simulink model "SimulacionTanque2"  (R2020a)
settings: Solver=VariableStepAuto  StartTime=0.0  StopTime=tsim  RelTol=1e-3
values from neighbouring files (symbols this model uses):
  tmuestra = 0.5    [GeneracionDatosTanque.m]    (also in LQRTanque.m; SimulacionTanque.m)
  tvar1 = 23    [GeneracionDatosTanque.m]    (also in SimulacionTanque.m)
  tvar2 = 24    [GeneracionDatosTanque.m]    (also in SimulacionTanque.m)
undefined symbols (not defined in the file or in its folder): alpha, Area, K1, K2, Kp, T1, T2, tau1, tau2, tdelay1, tdelay2, tdelayQ, Te
settings Model: Creator=pablo  LastModifiedBy=pablo
settings DataIOCC: SaveOutput=off  SignalLogging=off  DSMLogging=off  SaveTime=off  ReturnWorkspaceOutputs=off
settings DebuggingCC: ArithmeticOperatorsInVariantConditions=warning
settings SFSimCC: CustomCodeUndefinedFunction=UseInterfaceOnly

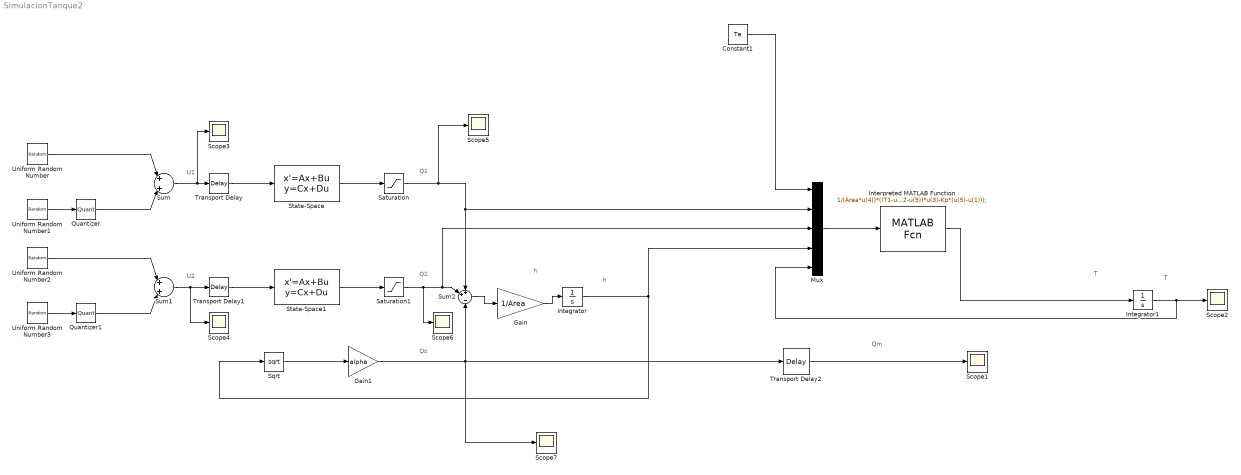
== system SimulacionTanque2 ==
  note: Qm
  note: .
      | T
  note: T
  note: h
  note: .
      |  h
  note: Qs
  note: Q1
  note: U1
  note: Q2
  note: U2
  Constant1 : Constant  Value=Te
  Gain : Gain  Gain=1/Area
  Gain1 : Gain  Gain=alpha
  Integrator : Integrator  InitialCondition=(4/alpha^2)  LimitOutput=on  LowerSaturationLimit=0
  Integrator1 : Integrator  InitialCondition=49.9  LowerSaturationLimit=0
  Interpreted MATLAB Function : MATLABFcn  MATLABFcn=1/(Area*u(4))*((T1-u(5))*u(2)+(T2-u(5))*u(3)-Kp*(u(5)-u(1)));  OutputDimensions=1
  Mux : Mux  Inputs=5
  Quantizer : Quantizer  QuantizationInterval=.25
  Quantizer1 : Quantizer  QuantizationInterval=.25
  Saturation : Saturate  UpperLimit=inf  LowerLimit=0
  Saturation1 : Saturate  UpperLimit=inf  LowerLimit=0
  Scope{1..7} (7 alike) : Scope
  Sqrt : Sqrt  SaturateOnIntegerOverflow=on
  State-Space : StateSpace  A=-1/tau1  B=K1/tau1  D=0  InitialCondition=2
  State-Space1 : StateSpace  A=-1/tau2  B=K2/tau2  D=0  InitialCondition=2
  Sum : Sum  Inputs=|+|+|
  Sum1 : Sum  Inputs=|+|+|
  Sum2 : Sum  Inputs=++|-
  Transport Delay : TransportDelay  DelayTime=tdelay1  InitialOutput=2
  Transport Delay1 : TransportDelay  DelayTime=tdelay2  InitialOutput=2
  Transport Delay2 : TransportDelay  DelayTime=tdelayQ  InitialOutput=4
  Uniform Random Number : UniformRandomNumber  Minimum=-.25  Maximum=.25  Seed=12378  SampleTime=tmuestra
  Uniform Random Number1 : UniformRandomNumber  Minimum=.125  Maximum=3.875  Seed=1008908  SampleTime=tvar1
  Uniform Random Number2 : UniformRandomNumber  Minimum=-.25  Maximum=.25  Seed=1239636  SampleTime=tmuestra
  Uniform Random Number3 : UniformRandomNumber  Minimum=.125  Maximum=3.875  Seed=5635694  SampleTime=tvar2
  wires:
  Uniform Random Number1/1 -> Quantizer/1
  Uniform Random Number/1 -> Sum/1
  Quantizer/1 -> Sum/2
  Sum/1 -> Scope3/1, Transport Delay/1
  Transport Delay/1 -> State-Space/1
  State-Space/1 -> Saturation/1
  Quantizer1/1 -> Sum1/2
  Transport Delay1/1 -> State-Space1/1
  Uniform Random Number3/1 -> Quantizer1/1
  State-Space1/1 -> Saturation1/1
  Sum1/1 -> Scope4/1, Transport Delay1/1
  Uniform Random Number2/1 -> Sum1/1
  Sum2/1 -> Gain/1
  Gain1/1 -> Scope7/1, Sum2/3, Transport Delay2/1
  Sqrt/1 -> Gain1/1
  Gain/1 -> Integrator/1
  Integrator/1 -> Sqrt/1, Mux/4
  Saturation/1 -> Scope5/1, Mux/2, Sum2/1
  Saturation1/1 -> Scope6/1, Mux/3, Sum2/2
  Constant1/1 -> Mux/1
  Integrator1/1 -> Mux/5, Scope2/1
  Interpreted MATLAB Function/1 -> Integrator1/1
  Transport Delay2/1 -> Scope1/1
  Mux/1 -> Interpreted MATLAB Function/1
